simulink model "sm_import_robot_stepfiles"  (R2020b)
settings: Solver=ode45  StartTime=0.0  StopTime=20  RelTol=1e-3  EnableMultiTasking=on
undefined symbols (not defined in the file): sigbuilder_block, X, Y, Z
libraries: sm_lib x49, nesl_utility x7
(part 2 of 2)

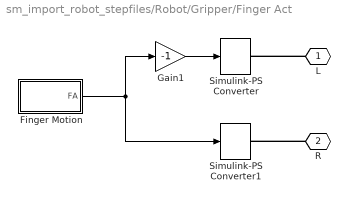
== system sm_import_robot_stepfiles/Robot/Gripper/Finger Act ==
  Finger Motion : Subsystem  Tag=STV Subsys  LoadFcn=sigbuilder_block('load');  StartFcn=sigbuilder_block('start');  StopFcn=sigbuilder_block('stop');  ClipboardFcn=sigbuilder_block('clipboard');  mask(Sigbuilder block){tuvar=[0:10]}
      mask help: Simulink:masks:SigbuilderBlock_MD
      mask init:
      | if ~strcmp(get_param(bdroot(gcbh),'SimulationStatus'),'stopped') tuvar = sigbuilder_block('maskInit'); end
      settings: CopyFcn=sigbuilder_block('copy');  DeleteFcn=sigbuilder_block('delete');  ModelCloseFcn=sigbuilder_block('modelClose');  PreSaveFcn=sigbuilder_block('preSave');  PauseFcn=sigbuilder_block('pause');  ContinueFcn=sigbuilder_block('continue');  NameChangeFcn=sigbuilder_block('namechange');  OpenFcn=sigbuilder_block('open',[437.6 199.2 550.4 400 ]);  CloseFcn=sigbuilder_block('close');
      mask Display: plot(0, 0, 100, 100,[2, 2, 32, 32, 2], [68, 8, 8, 68, 68],[32, 2], [38, 38], [32, 19, 2],[53, 60, 44], [32, 17, 17, 2],[16, 16, 31, 31]);txt = getActiveGroup(gcbh);text(2, 100, txt,'verticalAlignment', 'top');
  Gain1 : Gain  Gain=-1
  Simulink-PS Converter : nesl_utility/Simulink-PS Converter  PhysicalDomain=network_engine_domain  SubClassName=ps_input  LeftPortType=input  RightPortType=output  PseudoPeriodic=off  Frequencies=[]  NoiseDistribution=none  NoiseParameters=[]  Unit=deg  AffineConversion=off  FilteringAndDerivatives=filter  SimscapeFilterOrder=2  InputFilterTimeConstant=0.001  UdotUserProvided=1
      settings: SourceProductName=Utilities
  Simulink-PS Converter1 : nesl_utility/Simulink-PS Converter  PhysicalDomain=network_engine_domain  SubClassName=ps_input  LeftPortType=input  RightPortType=output  PseudoPeriodic=off  Frequencies=[]  NoiseDistribution=none  NoiseParameters=[]  Unit=deg  AffineConversion=off  FilteringAndDerivatives=filter  SimscapeFilterOrder=2  InputFilterTimeConstant=0.001  UdotUserProvided=1
      settings: SourceProductName=Utilities
  L : PMIOPort  Side=Right
  R : PMIOPort  Port=2  Side=Right
  wires:
  Finger Motion/1(FA) -> Simulink-PS Converter1/1, Gain1/1
  Gain1/1 -> Simulink-PS Converter/1
  connections:
  L/RConn1 -- Simulink-PS Converter/RConn1
  R/RConn1 -- Simulink-PS Converter1/RConn1

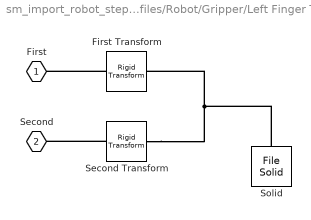
== system sm_import_robot_stepfiles/Robot/Gripper/Left Finger Tips ==
  First Transform : sm_lib/Frames and Transforms/Rigid Transform  TranslationMethod=Cartesian  TranslationStandardOffset=0  TranslationLengthUnit=cm  TranslationStandardAxis=+Z  TranslationCartesianOffset=[-2.5442152920324155 0.74021024484276698 0.82666565983828955]  TranslationROffset=0  TranslationROffsetUnits=m  TranslationZOffset=0  TranslationZOffsetUnits=m  TranslationThetaOffset=0  TranslationThetaOffsetUnits=deg  RotationMethod=ArbitraryAxis  RotationAngleUnits=deg  RotationStandardAxis=+Z  RotationAngle=120  RotationArbitraryAxis=[1 -1 1]  FollAlignAxisA=+X  BaseAlignAxisA=+Y  FollAlignAxisB=+Y  BaseAlignAxisB=+Z  RotationSequenceAxes=FollowerAxes  RotationSequence=XYX  RotationSequenceAngles=[0 0 0]  RotationSequenceAnglesUnits=deg  RotationMatrix=[1 0 0; 0 1 0; 0 0 1]
      settings: SourceProductName=Multibody
  Second Transform : sm_lib/Frames and Transforms/Rigid Transform  TranslationMethod=Cartesian  TranslationStandardOffset=0  TranslationLengthUnit=cm  TranslationStandardAxis=+Z  TranslationCartesianOffset=[-0.508 -0.61321024484276632 -0.2032]  TranslationROffset=0  TranslationROffsetUnits=m  TranslationZOffset=0  TranslationZOffsetUnits=m  TranslationThetaOffset=0  TranslationThetaOffsetUnits=deg  RotationMethod=ArbitraryAxis  RotationAngleUnits=deg  RotationStandardAxis=+Z  RotationAngle=120  RotationArbitraryAxis=[-1 -1 -1]  FollAlignAxisA=+X  BaseAlignAxisA=+Y  FollAlignAxisB=+Y  BaseAlignAxisB=+Z  RotationSequenceAxes=FollowerAxes  RotationSequence=XYX  RotationSequenceAngles=[0 0 0]  RotationSequenceAnglesUnits=deg  RotationMatrix=[1 0 0; 0 1 0; 0 0 1]
      settings: SourceProductName=Multibody
  Solid : sm_lib/Body Elements/File Solid  ExtGeomFileName=sm_srobot_fingertips.step  UnitType=FromFile  ExtGeomFileUnits=cm  StepReaderType=OCC  ExportConvexHullGeometry=off  InertiaType=CalculateFromGeometry  Mass=0.025178123679146753  MassUnits=kg  CenterOfMass=[0.28569571896451468 -5.4578424046040067e-05 0.069036811438125095]  CenterOfMassUnits=cm  MomentsOfInertia=[0.0065444380491917675 0.049015093978220708 0.046494149823922123]  MomentsOfInertiaUnits=kg*cm^2  ProductsOfInertia=[1.4396383276680692e-06 0.01060495039373101 -3.3718497055589141e-06]  ProductsOfInertiaUnits=kg*cm^2  BasedOnType=Mass  Density=1000  DensityUnits=kg/(m^3)  DoExposeReferenceFrame=on  SerializedFrames=<Frames/>  GraphicType=FromGeometry  MarkerShape=Sphere  MarkerSize=10  MarkerSizeUnits=m  GraphicVisPropType=SimpleVisualProperties  GraphicDiffuseColor=[0.47450980392156861 0.73725490196078436 1]  GraphicSpecularColor=[0.5 0.5 0.5 1.0]  GraphicAmbientColor=[0.15 0.15 0.15 1.0]  GraphicEmissiveColor=[0.0 0.0 0.0 1.0]  GraphicShininess=75  GraphicOpacity=1
      settings: SourceProductName=Multibody
  First : PMIOPort  Side=Left
  Second : PMIOPort  Port=2  Side=Left
  connections:
  Second Transform/LConn1 -- Solid/RConn1 -- First Transform/LConn1
  Second Transform/RConn1 -- Second/RConn1
  First Transform/RConn1 -- First/RConn1

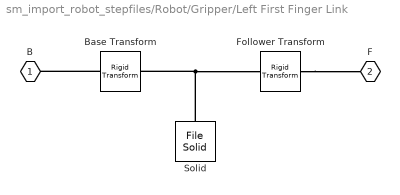
== system sm_import_robot_stepfiles/Robot/Gripper/Left First Finger Link ==
  Base Transform : sm_lib/Frames and Transforms/Rigid Transform  TranslationMethod=Cartesian  TranslationStandardOffset=0  TranslationLengthUnit=cm  TranslationStandardAxis=+Z  TranslationCartesianOffset=[0 -0.91801024484276572 0]  TranslationROffset=0  TranslationROffsetUnits=m  TranslationZOffset=0  TranslationZOffsetUnits=m  TranslationThetaOffset=0  TranslationThetaOffsetUnits=deg  RotationMethod=ArbitraryAxis  RotationAngleUnits=deg  RotationStandardAxis=+Z  RotationAngle=120  RotationArbitraryAxis=[-1 -1 -1]  FollAlignAxisA=+X  BaseAlignAxisA=+Y  FollAlignAxisB=+Y  BaseAlignAxisB=+Z  RotationSequenceAxes=FollowerAxes  RotationSequence=XYX  RotationSequenceAngles=[0 0 0]  RotationSequenceAnglesUnits=deg  RotationMatrix=[1 0 0; 0 1 0; 0 0 1]
      settings: SourceProductName=Multibody
  Follower Transform : sm_lib/Frames and Transforms/Rigid Transform  TranslationMethod=Cartesian  TranslationStandardOffset=0  TranslationLengthUnit=cm  TranslationStandardAxis=+Z  TranslationCartesianOffset=[1.778 -0.74021024484276632 -0.381]  TranslationROffset=0  TranslationROffsetUnits=m  TranslationZOffset=0  TranslationZOffsetUnits=m  TranslationThetaOffset=0  TranslationThetaOffsetUnits=deg  RotationMethod=ArbitraryAxis  RotationAngleUnits=deg  RotationStandardAxis=+Z  RotationAngle=120  RotationArbitraryAxis=[-1 -1 -1]  FollAlignAxisA=+X  BaseAlignAxisA=+Y  FollAlignAxisB=+Y  BaseAlignAxisB=+Z  RotationSequenceAxes=FollowerAxes  RotationSequence=XYX  RotationSequenceAngles=[0 0 0]  RotationSequenceAnglesUnits=deg  RotationMatrix=[1 0 0; 0 1 0; 0 0 1]
      settings: SourceProductName=Multibody
  Solid : sm_lib/Body Elements/File Solid  ExtGeomFileName=sm_srobot_lfirstfingerlink.step  UnitType=FromFile  ExtGeomFileUnits=cm  StepReaderType=OCC  ExportConvexHullGeometry=off  InertiaType=CalculateFromGeometry  Mass=0.0072753373091361435  MassUnits=kg  CenterOfMass=[0.57939854775507604 -0.065566988422878308 -0.41046090926561368]  CenterOfMassUnits=cm  MomentsOfInertia=[0.0013879268984117842 0.0054293039247647534 0.0057606720417102244]  MomentsOfInertiaUnits=kg*cm^2  ProductsOfInertia=[9.6984154429162483e-05 0.00030547405020594289 -0.00028824798134537063]  ProductsOfInertiaUnits=kg*cm^2  BasedOnType=Mass  Density=1000  DensityUnits=kg/(m^3)  DoExposeReferenceFrame=on  SerializedFrames=<Frames/>  GraphicType=FromGeometry  MarkerShape=Sphere  MarkerSize=10  MarkerSizeUnits=m  GraphicVisPropType=SimpleVisualProperties  GraphicDiffuseColor=[1 1 0.5490196078431373]  GraphicSpecularColor=[0.5 0.5 0.5 1.0]  GraphicAmbientColor=[0.15 0.15 0.15 1.0]  GraphicEmissiveColor=[0.0 0.0 0.0 1.0]  GraphicShininess=75  GraphicOpacity=1
      settings: SourceProductName=Multibody
  B : PMIOPort  Side=Left
  F : PMIOPort  Port=2  Side=Right
  connections:
  Solid/RConn1 -- Follower Transform/LConn1 -- Base Transform/LConn1
  Base Transform/RConn1 -- B/RConn1
  Follower Transform/RConn1 -- F/RConn1

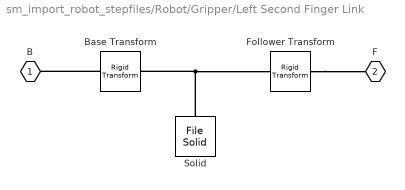
== system sm_import_robot_stepfiles/Robot/Gripper/Left Second Finger Link ==
  Base Transform : sm_lib/Frames and Transforms/Rigid Transform  TranslationMethod=Cartesian  TranslationStandardOffset=0  TranslationLengthUnit=cm  TranslationStandardAxis=+Z  TranslationCartesianOffset=[2.1844 -0.91801024484276572 0]  TranslationROffset=0  TranslationROffsetUnits=m  TranslationZOffset=0  TranslationZOffsetUnits=m  TranslationThetaOffset=0  TranslationThetaOffsetUnits=deg  RotationMethod=ArbitraryAxis  RotationAngleUnits=deg  RotationStandardAxis=+Z  RotationAngle=120  RotationArbitraryAxis=[-1 -1 -1]  FollAlignAxisA=+X  BaseAlignAxisA=+Y  FollAlignAxisB=+Y  BaseAlignAxisB=+Z  RotationSequenceAxes=FollowerAxes  RotationSequence=XYX  RotationSequenceAngles=[0 0 0]  RotationSequenceAnglesUnits=deg  RotationMatrix=[1 0 0; 0 1 0; 0 0 1]
      settings: SourceProductName=Multibody
  Follower Transform : sm_lib/Frames and Transforms/Rigid Transform  TranslationMethod=Cartesian  TranslationStandardOffset=0  TranslationLengthUnit=cm  TranslationStandardAxis=+Z  TranslationCartesianOffset=[0 0.61321024484276632 0]  TranslationROffset=0  TranslationROffsetUnits=m  TranslationZOffset=0  TranslationZOffsetUnits=m  TranslationThetaOffset=0  TranslationThetaOffsetUnits=deg  RotationMethod=ArbitraryAxis  RotationAngleUnits=deg  RotationStandardAxis=+Z  RotationAngle=120  RotationArbitraryAxis=[1 -1 1]  FollAlignAxisA=+X  BaseAlignAxisA=+Y  FollAlignAxisB=+Y  BaseAlignAxisB=+Z  RotationSequenceAxes=FollowerAxes  RotationSequence=XYX  RotationSequenceAngles=[0 0 0]  RotationSequenceAnglesUnits=deg  RotationMatrix=[1 0 0; 0 1 0; 0 0 1]
      settings: SourceProductName=Multibody
  Solid : sm_lib/Body Elements/File Solid  ExtGeomFileName=sm_srobot_secondfingerlink.step  UnitType=FromFile  ExtGeomFileUnits=cm  StepReaderType=OCC  ExportConvexHullGeometry=off  InertiaType=CalculateFromGeometry  Mass=0.005347817964666832  MassUnits=kg  CenterOfMass=[1.3095387695944416 0 0]  CenterOfMassUnits=cm  MomentsOfInertia=[0.00062632050801362594 0.0042402045040431545 0.0044495724115703027]  MomentsOfInertiaUnits=kg*cm^2  ProductsOfInertia=[0 0 0]  ProductsOfInertiaUnits=kg*cm^2  BasedOnType=Mass  Density=1000  DensityUnits=kg/(m^3)  DoExposeReferenceFrame=on  SerializedFrames=<Frames/>  GraphicType=FromGeometry  MarkerShape=Sphere  MarkerSize=10  MarkerSizeUnits=m  GraphicVisPropType=SimpleVisualProperties  GraphicDiffuseColor=[1 0 0]  GraphicSpecularColor=[0.5 0.5 0.5 1.0]  GraphicAmbientColor=[0.15 0.15 0.15 1.0]  GraphicEmissiveColor=[0.0 0.0 0.0 1.0]  GraphicShininess=75  GraphicOpacity=1
      settings: SourceProductName=Multibody
  B : PMIOPort  Side=Left
  F : PMIOPort  Port=2  Side=Right
  connections:
  Solid/RConn1 -- Base Transform/LConn1 -- Follower Transform/LConn1
  Base Transform/RConn1 -- B/RConn1
  Follower Transform/RConn1 -- F/RConn1

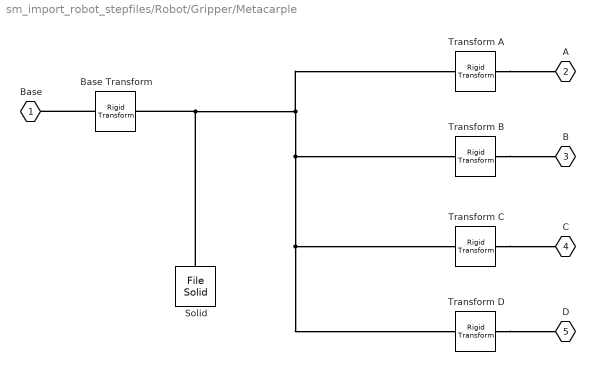
== system sm_import_robot_stepfiles/Robot/Gripper/Metacarple ==
  Base Transform : sm_lib/Frames and Transforms/Rigid Transform  TranslationMethod=Cartesian  TranslationStandardOffset=0  TranslationLengthUnit=cm  TranslationStandardAxis=+Z  TranslationCartesianOffset=[-1.27 0 0]  TranslationROffset=0  TranslationROffsetUnits=m  TranslationZOffset=0  TranslationZOffsetUnits=m  TranslationThetaOffset=0  TranslationThetaOffsetUnits=deg  RotationMethod=ArbitraryAxis  RotationAngleUnits=deg  RotationStandardAxis=+Z  RotationAngle=120  RotationArbitraryAxis=[-1 -1 1]  FollAlignAxisA=+X  BaseAlignAxisA=+Y  FollAlignAxisB=+Y  BaseAlignAxisB=+Z  RotationSequenceAxes=FollowerAxes  RotationSequence=XYX  RotationSequenceAngles=[0 0 0]  RotationSequenceAnglesUnits=deg  RotationMatrix=[1 0 0; 0 1 0; 0 0 1]
      settings: SourceProductName=Multibody
  Solid : sm_lib/Body Elements/File Solid  ExtGeomFileName=sm_srobot_metacarples.step  UnitType=FromFile  ExtGeomFileUnits=cm  StepReaderType=OCC  ExportConvexHullGeometry=off  InertiaType=CalculateFromGeometry  Mass=0.2949697962727843  MassUnits=kg  CenterOfMass=[0.51853214693243821 -2.1099755536633642e-07 1.2556451003194651e-07]  CenterOfMassUnits=cm  MomentsOfInertia=[0.78710657037075882 0.85556914968787445 0.70502786812617768]  MomentsOfInertiaUnits=kg*cm^2  ProductsOfInertia=[-8.2010371922616861e-08 1.5884273115413992e-07 1.1530290569471579e-07]  ProductsOfInertiaUnits=kg*cm^2  BasedOnType=Mass  Density=1000  DensityUnits=kg/(m^3)  DoExposeReferenceFrame=on  SerializedFrames=<Frames/>  GraphicType=FromGeometry  MarkerShape=Sphere  MarkerSize=10  MarkerSizeUnits=m  GraphicVisPropType=SimpleVisualProperties  GraphicDiffuseColor=[0.6588235294117647 1 0.82745098039215681]  GraphicSpecularColor=[0.5 0.5 0.5 1.0]  GraphicAmbientColor=[0.15 0.15 0.15 1.0]  GraphicEmissiveColor=[0.0 0.0 0.0 1.0]  GraphicShininess=75  GraphicOpacity=1
      settings: SourceProductName=Multibody
  Transform A : sm_lib/Frames and Transforms/Rigid Transform  TranslationMethod=Cartesian  TranslationStandardOffset=0  TranslationLengthUnit=cm  TranslationStandardAxis=+Z  TranslationCartesianOffset=[1.6022 -0.91801024484276572 -1.1156]  TranslationROffset=0  TranslationROffsetUnits=m  TranslationZOffset=0  TranslationZOffsetUnits=m  TranslationThetaOffset=0  TranslationThetaOffsetUnits=deg  RotationMethod=ArbitraryAxis  RotationAngleUnits=deg  RotationStandardAxis=+Z  RotationAngle=120  RotationArbitraryAxis=[-1 -1 -1]  FollAlignAxisA=+X  BaseAlignAxisA=+Y  FollAlignAxisB=+Y  BaseAlignAxisB=+Z  RotationSequenceAxes=FollowerAxes  RotationSequence=XYX  RotationSequenceAngles=[0 0 0]  RotationSequenceAnglesUnits=deg  RotationMatrix=[1 0 0; 0 1 0; 0 0 1]
      settings: SourceProductName=Multibody
  Transform B : sm_lib/Frames and Transforms/Rigid Transform  TranslationMethod=Cartesian  TranslationStandardOffset=0  TranslationLengthUnit=cm  TranslationStandardAxis=+Z  TranslationCartesianOffset=[3.6475045256124723 -0.9180102448427655 -0.54883545692650082]  TranslationROffset=0  TranslationROffsetUnits=m  TranslationZOffset=0  TranslationZOffsetUnits=m  TranslationThetaOffset=0  TranslationThetaOffsetUnits=deg  RotationMethod=ArbitraryAxis  RotationAngleUnits=deg  RotationStandardAxis=+Z  RotationAngle=120  RotationArbitraryAxis=[-1 -1 -1]  FollAlignAxisA=+X  BaseAlignAxisA=+Y  FollAlignAxisB=+Y  BaseAlignAxisB=+Z  RotationSequenceAxes=FollowerAxes  RotationSequence=XYX  RotationSequenceAngles=[0 0 0]  RotationSequenceAnglesUnits=deg  RotationMatrix=[1 0 0; 0 1 0; 0 0 1]
      settings: SourceProductName=Multibody
  Transform C : sm_lib/Frames and Transforms/Rigid Transform  TranslationMethod=Cartesian  TranslationStandardOffset=0  TranslationLengthUnit=cm  TranslationStandardAxis=+Z  TranslationCartesianOffset=[3.6475045256124723 -0.9180102448427655 0.54883545692650082]  TranslationROffset=0  TranslationROffsetUnits=m  TranslationZOffset=0  TranslationZOffsetUnits=m  TranslationThetaOffset=0  TranslationThetaOffsetUnits=deg  RotationMethod=ArbitraryAxis  RotationAngleUnits=deg  RotationStandardAxis=+Z  RotationAngle=120  RotationArbitraryAxis=[-1 -1 -1]  FollAlignAxisA=+X  BaseAlignAxisA=+Y  FollAlignAxisB=+Y  BaseAlignAxisB=+Z  RotationSequenceAxes=FollowerAxes  RotationSequence=XYX  RotationSequenceAngles=[0 0 0]  RotationSequenceAnglesUnits=deg  RotationMatrix=[1 0 0; 0 1 0; 0 0 1]
      settings: SourceProductName=Multibody
  Transform D : sm_lib/Frames and Transforms/Rigid Transform  TranslationMethod=Cartesian  TranslationStandardOffset=0  TranslationLengthUnit=cm  TranslationStandardAxis=+Z  TranslationCartesianOffset=[1.6022 -0.91801024484276572 1.1156]  TranslationROffset=0  TranslationROffsetUnits=m  TranslationZOffset=0  TranslationZOffsetUnits=m  TranslationThetaOffset=0  TranslationThetaOffsetUnits=deg  RotationMethod=ArbitraryAxis  RotationAngleUnits=deg  RotationStandardAxis=+Z  RotationAngle=120  RotationArbitraryAxis=[-1 -1 -1]  FollAlignAxisA=+X  BaseAlignAxisA=+Y  FollAlignAxisB=+Y  BaseAlignAxisB=+Z  RotationSequenceAxes=FollowerAxes  RotationSequence=XYX  RotationSequenceAngles=[0 0 0]  RotationSequenceAnglesUnits=deg  RotationMatrix=[1 0 0; 0 1 0; 0 0 1]
      settings: SourceProductName=Multibody
  Base : PMIOPort  Side=Left
  A : PMIOPort  Port=2  Side=Right
  B : PMIOPort  Port=3  Side=Right
  C : PMIOPort  Port=4  Side=Right
  D : PMIOPort  Port=5  Side=Right
  connections:
  Solid/RConn1 -- Base Transform/LConn1 -- Transform D/LConn1 -- Transform C/LConn1 -- Transform B/LConn1 -- Transform A/LConn1
  Transform D/RConn1 -- D/RConn1
  Transform C/RConn1 -- C/RConn1
  Transform B/RConn1 -- B/RConn1
  Transform A/RConn1 -- A/RConn1
  Base Transform/RConn1 -- Base/RConn1

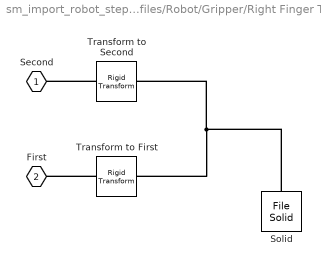
== system sm_import_robot_stepfiles/Robot/Gripper/Right Finger Tips ==
  Solid : sm_lib/Body Elements/File Solid  ExtGeomFileName=sm_srobot_fingertips.step  UnitType=FromFile  ExtGeomFileUnits=cm  StepReaderType=OCC  ExportConvexHullGeometry=off  InertiaType=CalculateFromGeometry  Mass=0.025178123679146753  MassUnits=kg  CenterOfMass=[0.28569571896451468 -5.4578424046040067e-05 0.069036811438125095]  CenterOfMassUnits=cm  MomentsOfInertia=[0.0065444380491917675 0.049015093978220708 0.046494149823922123]  MomentsOfInertiaUnits=kg*cm^2  ProductsOfInertia=[1.4396383276680692e-06 0.01060495039373101 -3.3718497055589141e-06]  ProductsOfInertiaUnits=kg*cm^2  BasedOnType=Mass  Density=1000  DensityUnits=kg/(m^3)  DoExposeReferenceFrame=on  SerializedFrames=<Frames/>  GraphicType=FromGeometry  MarkerShape=Sphere  MarkerSize=10  MarkerSizeUnits=m  GraphicVisPropType=SimpleVisualProperties  GraphicDiffuseColor=[0.47450980392156861 0.73725490196078436 1]  GraphicSpecularColor=[0.5 0.5 0.5 1.0]  GraphicAmbientColor=[0.15 0.15 0.15 1.0]  GraphicEmissiveColor=[0.0 0.0 0.0 1.0]  GraphicShininess=75  GraphicOpacity=1
      settings: SourceProductName=Multibody
  Transform to First : sm_lib/Frames and Transforms/Rigid Transform  TranslationMethod=Cartesian  TranslationStandardOffset=0  TranslationLengthUnit=cm  TranslationStandardAxis=+Z  TranslationCartesianOffset=[-2.544215292032415 -0.74021024484276632 0.82666565983828855]  TranslationROffset=0  TranslationROffsetUnits=m  TranslationZOffset=0  TranslationZOffsetUnits=m  TranslationThetaOffset=0  TranslationThetaOffsetUnits=deg  RotationMethod=ArbitraryAxis  RotationAngleUnits=deg  RotationStandardAxis=+Z  RotationAngle=120  RotationArbitraryAxis=[-1 -1 -1]  FollAlignAxisA=+X  BaseAlignAxisA=+Y  FollAlignAxisB=+Y  BaseAlignAxisB=+Z  RotationSequenceAxes=FollowerAxes  RotationSequence=XYX  RotationSequenceAngles=[0 0 0]  RotationSequenceAnglesUnits=deg  RotationMatrix=[1 0 0; 0 1 0; 0 0 1]
      settings: SourceProductName=Multibody
  Transform to Second : sm_lib/Frames and Transforms/Rigid Transform  TranslationMethod=Cartesian  TranslationStandardOffset=0  TranslationLengthUnit=cm  TranslationStandardAxis=+Z  TranslationCartesianOffset=[-0.508 0.61321024484276621 -0.2032]  TranslationROffset=0  TranslationROffsetUnits=m  TranslationZOffset=0  TranslationZOffsetUnits=m  TranslationThetaOffset=0  TranslationThetaOffsetUnits=deg  RotationMethod=ArbitraryAxis  RotationAngleUnits=deg  RotationStandardAxis=+Z  RotationAngle=120  RotationArbitraryAxis=[1 -1 1]  FollAlignAxisA=+X  BaseAlignAxisA=+Y  FollAlignAxisB=+Y  BaseAlignAxisB=+Z  RotationSequenceAxes=FollowerAxes  RotationSequence=XYX  RotationSequenceAngles=[0 0 0]  RotationSequenceAnglesUnits=deg  RotationMatrix=[1 0 0; 0 1 0; 0 0 1]
      settings: SourceProductName=Multibody
  Second : PMIOPort  Side=Left
  First : PMIOPort  Port=2  Side=Left
  connections:
  Solid/RConn1 -- Transform to Second/LConn1 -- Transform to First/LConn1
  Transform to First/RConn1 -- First/RConn1
  Transform to Second/RConn1 -- Second/RConn1

== system sm_import_robot_stepfiles/Robot/Gripper/Right First Finger Link ==
  Base Transform : sm_lib/Frames and Transforms/Rigid Transform  TranslationMethod=Cartesian  TranslationStandardOffset=0  TranslationLengthUnit=cm  TranslationStandardAxis=+Z  TranslationCartesianOffset=[0 -0.91801024484276572 0]  TranslationROffset=0  TranslationROffsetUnits=m  TranslationZOffset=0  TranslationZOffsetUnits=m  TranslationThetaOffset=0  TranslationThetaOffsetUnits=deg  RotationMethod=ArbitraryAxis  RotationAngleUnits=deg  RotationStandardAxis=+Z  RotationAngle=120  RotationArbitraryAxis=[-1 -1 -1]  FollAlignAxisA=+X  BaseAlignAxisA=+Y  FollAlignAxisB=+Y  BaseAlignAxisB=+Z  RotationSequenceAxes=FollowerAxes  RotationSequence=XYX  RotationSequenceAngles=[0 0 0]  RotationSequenceAnglesUnits=deg  RotationMatrix=[1 0 0; 0 1 0; 0 0 1]
      settings: SourceProductName=Multibody
  Follower Transform : sm_lib/Frames and Transforms/Rigid Transform  TranslationMethod=Cartesian  TranslationStandardOffset=0  TranslationLengthUnit=cm  TranslationStandardAxis=+Z  TranslationCartesianOffset=[1.778 -0.74021024484276632 0.381]  TranslationROffset=0  TranslationROffsetUnits=m  TranslationZOffset=0  TranslationZOffsetUnits=m  TranslationThetaOffset=0  TranslationThetaOffsetUnits=deg  RotationMethod=ArbitraryAxis  RotationAngleUnits=deg  RotationStandardAxis=+Z  RotationAngle=120  RotationArbitraryAxis=[-1 -1 -1]  FollAlignAxisA=+X  BaseAlignAxisA=+Y  FollAlignAxisB=+Y  BaseAlignAxisB=+Z  RotationSequenceAxes=FollowerAxes  RotationSequence=XYX  RotationSequenceAngles=[0 0 0]  RotationSequenceAnglesUnits=deg  RotationMatrix=[1 0 0; 0 1 0; 0 0 1]
      settings: SourceProductName=Multibody
  Solid : sm_lib/Body Elements/File Solid  ExtGeomFileName=sm_srobot_rfirstfingerlink.step  UnitType=FromFile  ExtGeomFileUnits=cm  StepReaderType=OCC  ExportConvexHullGeometry=off  InertiaType=CalculateFromGeometry  Mass=0.0072753633395043153  MassUnits=kg  CenterOfMass=[0.5793957104083951 -0.065568525374514061 0.41045924650847537]  CenterOfMassUnits=cm  MomentsOfInertia=[0.0013879360712697633 0.0054293297573781941 0.0057606953913205416]  MomentsOfInertiaUnits=kg*cm^2  ProductsOfInertia=[-9.6988344798463436e-05 -0.00030548455416942526 -0.00028825710364633017]  ProductsOfInertiaUnits=kg*cm^2  BasedOnType=Mass  Density=1000  DensityUnits=kg/(m^3)  DoExposeReferenceFrame=on  SerializedFrames=<Frames/>  GraphicType=FromGeometry  MarkerShape=Sphere  MarkerSize=10  MarkerSizeUnits=m  GraphicVisPropType=SimpleVisualProperties  GraphicDiffuseColor=[1 1 0.5490196078431373]  GraphicSpecularColor=[0.5 0.5 0.5 1.0]  GraphicAmbientColor=[0.15 0.15 0.15 1.0]  GraphicEmissiveColor=[0.0 0.0 0.0 1.0]  GraphicShininess=75  GraphicOpacity=1
      settings: SourceProductName=Multibody
  B : PMIOPort  Side=Left
  F : PMIOPort  Port=2  Side=Right
  connections:
  Solid/RConn1 -- Base Transform/LConn1 -- Follower Transform/LConn1
  Base Transform/RConn1 -- B/RConn1
  Follower Transform/RConn1 -- F/RConn1

== system sm_import_robot_stepfiles/Robot/Gripper/Right Second Finger Link ==
  Base Transform : sm_lib/Frames and Transforms/Rigid Transform  TranslationMethod=Cartesian  TranslationStandardOffset=0  TranslationLengthUnit=cm  TranslationStandardAxis=+Z  TranslationCartesianOffset=[2.1844 -0.91801024484276539 0]  TranslationROffset=0  TranslationROffsetUnits=m  TranslationZOffset=0  TranslationZOffsetUnits=m  TranslationThetaOffset=0  TranslationThetaOffsetUnits=deg  RotationMethod=ArbitraryAxis  RotationAngleUnits=deg  RotationStandardAxis=+Z  RotationAngle=120  RotationArbitraryAxis=[-1 -1 -1]  FollAlignAxisA=+X  BaseAlignAxisA=+Y  FollAlignAxisB=+Y  BaseAlignAxisB=+Z  RotationSequenceAxes=FollowerAxes  RotationSequence=XYX  RotationSequenceAngles=[0 0 0]  RotationSequenceAnglesUnits=deg  RotationMatrix=[1 0 0; 0 1 0; 0 0 1]
      settings: SourceProductName=Multibody
  Follower Transform : sm_lib/Frames and Transforms/Rigid Transform  TranslationMethod=Cartesian  TranslationStandardOffset=0  TranslationLengthUnit=cm  TranslationStandardAxis=+Z  TranslationCartesianOffset=[0 0.61321024484276621 0]  TranslationROffset=0  TranslationROffsetUnits=m  TranslationZOffset=0  TranslationZOffsetUnits=m  TranslationThetaOffset=0  TranslationThetaOffsetUnits=deg  RotationMethod=ArbitraryAxis  RotationAngleUnits=deg  RotationStandardAxis=+Z  RotationAngle=120  RotationArbitraryAxis=[1 -1 1]  FollAlignAxisA=+X  BaseAlignAxisA=+Y  FollAlignAxisB=+Y  BaseAlignAxisB=+Z  RotationSequenceAxes=FollowerAxes  RotationSequence=XYX  RotationSequenceAngles=[0 0 0]  RotationSequenceAnglesUnits=deg  RotationMatrix=[1 0 0; 0 1 0; 0 0 1]
      settings: SourceProductName=Multibody
  Solid : sm_lib/Body Elements/File Solid  ExtGeomFileName=sm_srobot_secondfingerlink.step  UnitType=FromFile  ExtGeomFileUnits=cm  StepReaderType=OCC  ExportConvexHullGeometry=off  InertiaType=CalculateFromGeometry  Mass=0.005347817964666832  MassUnits=kg  CenterOfMass=[1.3095387695944416 0 0]  CenterOfMassUnits=cm  MomentsOfInertia=[0.00062632050801362594 0.0042402045040431545 0.0044495724115703027]  MomentsOfInertiaUnits=kg*cm^2  ProductsOfInertia=[0 0 0]  ProductsOfInertiaUnits=kg*cm^2  BasedOnType=Mass  Density=1000  DensityUnits=kg/(m^3)  DoExposeReferenceFrame=on  SerializedFrames=<Frames/>  GraphicType=FromGeometry  MarkerShape=Sphere  MarkerSize=10  MarkerSizeUnits=m  GraphicVisPropType=SimpleVisualProperties  GraphicDiffuseColor=[1 0 0]  GraphicSpecularColor=[0.5 0.5 0.5 1.0]  GraphicAmbientColor=[0.15 0.15 0.15 1.0]  GraphicEmissiveColor=[0.0 0.0 0.0 1.0]  GraphicShininess=75  GraphicOpacity=1
      settings: SourceProductName=Multibody
  B : PMIOPort  Side=Left
  F : PMIOPort  Port=2  Side=Right
  connections:
  Solid/RConn1 -- Follower Transform/LConn1 -- Base Transform/LConn1
  Base Transform/RConn1 -- B/RConn1
  Follower Transform/RConn1 -- F/RConn1

== system sm_import_robot_stepfiles/Robot/Gripper Actuation/Gripper Motion ==
  Demux : Demux  Tag=STV Demux  Outputs=1
      settings: DisplayOption=none
  FromWs : FromWorkspace  Tag=STV FromWs  VariableName=tuvar
      SigBuilderData=|
      | common.afterFinalStr = 'Extrapolate'
      | common.sampleTime = 0
      | dataSet.timeRange = [0 20]
      | dataSet.name = 'Motion'
      | sbobj.Groups.Name = 'Motion'
      | sbobj.Groups.Signals.Name = 'GA'
      | sbobj.Groups.Signals.XData = [0 2.5 4.5 5.5 7.5 12.5 14.5 15.5 17.5 20]
      | sbobj.Groups.Signals.YData = [0 0 45 45 0 0 -45 -45 0 0]
      | sbobj.Groups.TimeRange = [0 20]
  GA : Outport  Tag=STV Outport
  wires:
  Demux/1 -> GA/1
  FromWs/1 -> Demux/1

== system sm_import_robot_stepfiles/Robot/Upperarm Actuation/Upper Arm Motion ==
  Demux : Demux  Tag=STV Demux  Outputs=1
      settings: DisplayOption=none
  FromWs : FromWorkspace  Tag=STV FromWs  VariableName=tuvar
      SigBuilderData=|
      | common.afterFinalStr = 'Extrapolate'
      | common.sampleTime = 0
      | dataSet.timeRange = [0 20]
      | dataSet.name = 'Motion'
      | sbobj.Groups.Name = 'Motion'
      | sbobj.Groups.Signals.Name = 'UA'
      | sbobj.Groups.Signals.XData = [0 2.5 7.5 12.5 17.5 20]
      | sbobj.Groups.Signals.YData = [0 -90 -90 90 90 0]
      | sbobj.Groups.TimeRange = [0 20]
  UA : Outport  Tag=STV Outport
  wires:
  Demux/1 -> UA/1
  FromWs/1 -> Demux/1

== system sm_import_robot_stepfiles/Robot/Wrist Actuation/Wrist Motion ==
  Demux : Demux  Tag=STV Demux  Outputs=1
      settings: DisplayOption=none
  FromWs : FromWorkspace  Tag=STV FromWs  VariableName=tuvar
      SigBuilderData=|
      | common.afterFinalStr = 'Extrapolate'
      | common.sampleTime = 0
      | dataSet.timeRange = [0 20]
      | dataSet.name = 'Motion'
      | sbobj.Groups.Name = 'Motion'
      | sbobj.Groups.Signals.Name = 'WA'
      | sbobj.Groups.Signals.XData = [0 2.5 4.5 5.5 7.5 12.5 14.5 15.5 17.5 20]
      | sbobj.Groups.Signals.YData = [0 0 -90 -90 0 0 -90 -90 0 0]
      | sbobj.Groups.TimeRange = [0 20]
  WA : Outport  Tag=STV Outport
  wires:
  FromWs/1 -> Demux/1
  Demux/1 -> WA/1

== system sm_import_robot_stepfiles/Robot/Gripper/Finger Act/Finger Motion ==
  Demux : Demux  Tag=STV Demux  Outputs=1
      settings: DisplayOption=none
  FromWs : FromWorkspace  Tag=STV FromWs  VariableName=tuvar
      SigBuilderData=|
      | common.afterFinalStr = 'Extrapolate'
      | common.sampleTime = 0
      | dataSet.timeRange = [0 20]
      | dataSet.name = 'Motion'
      | sbobj.Groups.Name = 'Motion'
      | sbobj.Groups.Signals.Name = 'FA'
      | sbobj.Groups.Signals.XData = [0 4 4.5 5.5 6 14.5 15.5 20]
      | sbobj.Groups.Signals.YData = [130 130 130 150 150 150 130 130]
      | sbobj.Groups.TimeRange = [0 20]
  FA : Outport  Tag=STV Outport
  wires:
  Demux/1 -> FA/1
  FromWs/1 -> Demux/1
